simulink model "VCU_CS75_12_27_test"  (R2014a)
settings: Solver=FixedStepDiscrete  StartTime=0.0  StopTime=25  FixedStep=0.0005  RelTol=1e-3
undefined symbols (not defined in the file): D1, D2, D3, ecucoder_acal, ErrorSumMax1, ErrorSumMax2, ErrorSumMax3, I1, I2, I3, I_SW01_L, LaterlAngleCommand, LDW, P1, P2, P3, RemoteAcclPosition
libraries: simulink x913, ec5744lib x39
(part 19 of 30)

== system VCU_CS75_12_27_test/长安CS75底盘程序，20ms一次/Output/Subsystem/TransmitMessages1/ACC_34E/ACC_RLaneDistanceFusion ==
  ACC_RLaneDistanceFusion : Inport
  ACC_RLaneDistanceFusionBitCov : DataTypeConversion  OutDataTypeStr=uint8
  ACC_RLaneDistanceFusionCOV : DataTypeConversion  OutDataTypeStr=uint8
  ACC_RLaneDistanceFusionRon : Rounding  Operator=round
  ACC_RLaneDistanceFusion_1sat : Saturate  UpperLimit=1016  LowerLimit=0
  ACC_RLaneDistanceFusion_And : simulink/Logic and Bit Operations/Bitwise Operator  logicop=AND  UseBitMask=off  NumInputPorts=2  BitMask=bin2dec('11011001')  BitMaskRealWorld=Stored Integer
  ACC_RLaneDistanceFusion_And_C : Constant  Value=255  OutDataTypeStr=uint32
  ACC_RLaneDistanceFusion_Convert : DataTypeConversion  OutDataTypeStr=uint32
  ACC_RLaneDistanceFusion_D : Product  Inputs=*/
  ACC_RLaneDistanceFusion_D1 : Product  Inputs=*/
  ACC_RLaneDistanceFusion_F : Constant  Value=0.05  OutDataTypeStr=single
  ACC_RLaneDistanceFusion_L : simulink/Logic and Bit Operations/Bitwise Operator  logicop=AND  UseBitMask=on  BitMask=1016  BitMaskRealWorld=Stored Integer
  ACC_RLaneDistanceFusion_O : Constant  Value=0  OutDataTypeStr=single
  ACC_RLaneDistanceFusion_S : ArithShift  BitShiftNumber=-3
  ACC_RLaneDistanceFusion_sat : Saturate  UpperLimit=6.35  LowerLimit=0
  ACC_RLaneDistanceFusion_st : Sum  Inputs=+-
  ACC_RLaneDistanceFusionoutput2_C : Constant  Value=256
  Constant{1,4..8} (6 alike) : Constant  Value=0  OutDataTypeStr=uint8
  output1 : Outport
  output2 : Outport  Port=2
  output3 : Outport  Port=3
  output4 : Outport  Port=4
  output5 : Outport  Port=5
  output6 : Outport  Port=6
  output7 : Outport  Port=7
  output8 : Outport  Port=8
  wires:
  ACC_RLaneDistanceFusion/1 -> ACC_RLaneDistanceFusion_sat/1
  ACC_RLaneDistanceFusion_sat/1 -> ACC_RLaneDistanceFusion_st/1
  ACC_RLaneDistanceFusion_O/1 -> ACC_RLaneDistanceFusion_st/2
  ACC_RLaneDistanceFusion_st/1 -> ACC_RLaneDistanceFusion_D/1
  ACC_RLaneDistanceFusion_F/1 -> ACC_RLaneDistanceFusion_D/2
  ACC_RLaneDistanceFusion_D/1 -> ACC_RLaneDistanceFusionRon/1
  ACC_RLaneDistanceFusionRon/1 -> ACC_RLaneDistanceFusion_S/1
  ACC_RLaneDistanceFusion_S/1 -> ACC_RLaneDistanceFusion_1sat/1
  ACC_RLaneDistanceFusion_1sat/1 -> ACC_RLaneDistanceFusion_Convert/1
  ACC_RLaneDistanceFusion_Convert/1 -> ACC_RLaneDistanceFusion_L/1
  ACC_RLaneDistanceFusion_L/1 -> ACC_RLaneDistanceFusion_D1/1, ACC_RLaneDistanceFusion_And/1
  ACC_RLaneDistanceFusionoutput2_C/1 -> ACC_RLaneDistanceFusion_D1/2
  ACC_RLaneDistanceFusion_D1/1 -> ACC_RLaneDistanceFusionCOV/1
  ACC_RLaneDistanceFusionCOV/1 -> output2/1
  ACC_RLaneDistanceFusion_And_C/1 -> ACC_RLaneDistanceFusion_And/2
  ACC_RLaneDistanceFusion_And/1 -> ACC_RLaneDistanceFusionBitCov/1
  ACC_RLaneDistanceFusionBitCov/1 -> output3/1
  Constant1/1 -> output1/1
  Constant4/1 -> output4/1
  Constant5/1 -> output5/1
  Constant6/1 -> output6/1
  Constant7/1 -> output7/1
  Constant8/1 -> output8/1

== system VCU_CS75_12_27_test/长安CS75底盘程序，20ms一次/Output/Subsystem/TransmitMessages1/ACC_34E/ACC_RelevantTargetDection ==
  ACC_RelevantTargetDection : Inport
  ACC_RelevantTargetDectionRon : Rounding  Operator=round
  ACC_RelevantTargetDection_1sat : Saturate  UpperLimit=12  LowerLimit=0
  ACC_RelevantTargetDection_Convert : DataTypeConversion  OutDataTypeStr=uint8
  ACC_RelevantTargetDection_Convert1 : DataTypeConversion  OutDataTypeStr=uint32
  ACC_RelevantTargetDection_D : Product  Inputs=*/
  ACC_RelevantTargetDection_F : Constant  OutDataTypeStr=single
  ACC_RelevantTargetDection_L : simulink/Logic and Bit Operations/Bitwise Operator  logicop=AND  UseBitMask=on  BitMask=12  BitMaskRealWorld=Stored Integer
  ACC_RelevantTargetDection_O : Constant  Value=0  OutDataTypeStr=single
  ACC_RelevantTargetDection_S : ArithShift  BitShiftNumber=-2
  ACC_RelevantTargetDection_sat : Saturate  UpperLimit=3  LowerLimit=0
  ACC_RelevantTargetDection_st : Sum  Inputs=+-
  Constant{1,3..8} (7 alike) : Constant  Value=0  OutDataTypeStr=uint8
  output1 : Outport
  output2 : Outport  Port=2
  output3 : Outport  Port=3
  output4 : Outport  Port=4
  output5 : Outport  Port=5
  output6 : Outport  Port=6
  output7 : Outport  Port=7
  output8 : Outport  Port=8
  wires:
  ACC_RelevantTargetDection/1 -> ACC_RelevantTargetDection_sat/1
  ACC_RelevantTargetDection_sat/1 -> ACC_RelevantTargetDection_st/1
  ACC_RelevantTargetDection_O/1 -> ACC_RelevantTargetDection_st/2
  ACC_RelevantTargetDection_st/1 -> ACC_RelevantTargetDection_D/1
  ACC_RelevantTargetDection_F/1 -> ACC_RelevantTargetDection_D/2
  ACC_RelevantTargetDection_D/1 -> ACC_RelevantTargetDectionRon/1
  ACC_RelevantTargetDectionRon/1 -> ACC_RelevantTargetDection_S/1
  ACC_RelevantTargetDection_S/1 -> ACC_RelevantTargetDection_1sat/1
  ACC_RelevantTargetDection_1sat/1 -> ACC_RelevantTargetDection_Convert1/1
  ACC_RelevantTargetDection_Convert1/1 -> ACC_RelevantTargetDection_L/1
  ACC_RelevantTargetDection_L/1 -> ACC_RelevantTargetDection_Convert/1
  ACC_RelevantTargetDection_Convert/1 -> output2/1
  Constant1/1 -> output1/1
  Constant3/1 -> output3/1
  Constant4/1 -> output4/1
  Constant5/1 -> output5/1
  Constant6/1 -> output6/1
  Constant7/1 -> output7/1
  Constant8/1 -> output8/1

== system VCU_CS75_12_27_test/长安CS75底盘程序，20ms一次/Output/Subsystem/TransmitMessages1/ACC_34E/ACC_RelevantTargetID ==
  ACC_RelevantTargetID : Inport
  ACC_RelevantTargetIDRon : Rounding  Operator=round
  ACC_RelevantTargetID_1sat : Saturate  UpperLimit=240  LowerLimit=0
  ACC_RelevantTargetID_Convert : DataTypeConversion  OutDataTypeStr=uint8
  ACC_RelevantTargetID_Convert1 : DataTypeConversion  OutDataTypeStr=uint32
  ACC_RelevantTargetID_D : Product  Inputs=*/
  ACC_RelevantTargetID_F : Constant  OutDataTypeStr=single
  ACC_RelevantTargetID_L : simulink/Logic and Bit Operations/Bitwise Operator  logicop=AND  UseBitMask=on  BitMask=240  BitMaskRealWorld=Stored Integer
  ACC_RelevantTargetID_O : Constant  Value=0  OutDataTypeStr=single
  ACC_RelevantTargetID_S : ArithShift  BitShiftNumber=-4
  ACC_RelevantTargetID_sat : Saturate  UpperLimit=15  LowerLimit=0
  ACC_RelevantTargetID_st : Sum  Inputs=+-
  Constant{2..8} (7 alike) : Constant  Value=0  OutDataTypeStr=uint8
  output1 : Outport
  output2 : Outport  Port=2
  output3 : Outport  Port=3
  output4 : Outport  Port=4
  output5 : Outport  Port=5
  output6 : Outport  Port=6
  output7 : Outport  Port=7
  output8 : Outport  Port=8
  wires:
  ACC_RelevantTargetID/1 -> ACC_RelevantTargetID_sat/1
  ACC_RelevantTargetID_sat/1 -> ACC_RelevantTargetID_st/1
  ACC_RelevantTargetID_O/1 -> ACC_RelevantTargetID_st/2
  ACC_RelevantTargetID_st/1 -> ACC_RelevantTargetID_D/1
  ACC_RelevantTargetID_F/1 -> ACC_RelevantTargetID_D/2
  ACC_RelevantTargetID_D/1 -> ACC_RelevantTargetIDRon/1
  ACC_RelevantTargetIDRon/1 -> ACC_RelevantTargetID_S/1
  ACC_RelevantTargetID_S/1 -> ACC_RelevantTargetID_1sat/1
  ACC_RelevantTargetID_1sat/1 -> ACC_RelevantTargetID_Convert1/1
  ACC_RelevantTargetID_Convert1/1 -> ACC_RelevantTargetID_L/1
  ACC_RelevantTargetID_L/1 -> ACC_RelevantTargetID_Convert/1
  ACC_RelevantTargetID_Convert/1 -> output1/1
  Constant2/1 -> output2/1
  Constant3/1 -> output3/1
  Constant4/1 -> output4/1
  Constant5/1 -> output5/1
  Constant6/1 -> output6/1
  Constant7/1 -> output7/1
  Constant8/1 -> output8/1

== system VCU_CS75_12_27_test/长安CS75底盘程序，20ms一次/Output/Subsystem/TransmitMessages1/ACC_34E/ACC_RightTargetID ==
  ACC_RightTargetID : Inport
  ACC_RightTargetIDRon : Rounding  Operator=round
  ACC_RightTargetID_1sat : Saturate  UpperLimit=240  LowerLimit=0
  ACC_RightTargetID_Convert : DataTypeConversion  OutDataTypeStr=uint8
  ACC_RightTargetID_Convert1 : DataTypeConversion  OutDataTypeStr=uint32
  ACC_RightTargetID_D : Product  Inputs=*/
  ACC_RightTargetID_F : Constant  OutDataTypeStr=single
  ACC_RightTargetID_L : simulink/Logic and Bit Operations/Bitwise Operator  logicop=AND  UseBitMask=on  BitMask=240  BitMaskRealWorld=Stored Integer
  ACC_RightTargetID_O : Constant  Value=0  OutDataTypeStr=single
  ACC_RightTargetID_S : ArithShift  BitShiftNumber=-4
  ACC_RightTargetID_sat : Saturate  UpperLimit=15  LowerLimit=0
  ACC_RightTargetID_st : Sum  Inputs=+-
  Constant{1,3..8} (7 alike) : Constant  Value=0  OutDataTypeStr=uint8
  output1 : Outport
  output2 : Outport  Port=2
  output3 : Outport  Port=3
  output4 : Outport  Port=4
  output5 : Outport  Port=5
  output6 : Outport  Port=6
  output7 : Outport  Port=7
  output8 : Outport  Port=8
  wires:
  ACC_RightTargetID/1 -> ACC_RightTargetID_sat/1
  ACC_RightTargetID_sat/1 -> ACC_RightTargetID_st/1
  ACC_RightTargetID_O/1 -> ACC_RightTargetID_st/2
  ACC_RightTargetID_st/1 -> ACC_RightTargetID_D/1
  ACC_RightTargetID_F/1 -> ACC_RightTargetID_D/2
  ACC_RightTargetID_D/1 -> ACC_RightTargetIDRon/1
  ACC_RightTargetIDRon/1 -> ACC_RightTargetID_S/1
  ACC_RightTargetID_S/1 -> ACC_RightTargetID_1sat/1
  ACC_RightTargetID_1sat/1 -> ACC_RightTargetID_Convert1/1
  ACC_RightTargetID_Convert1/1 -> ACC_RightTargetID_L/1
  ACC_RightTargetID_L/1 -> ACC_RightTargetID_Convert/1
  ACC_RightTargetID_Convert/1 -> output2/1
  Constant1/1 -> output1/1
  Constant3/1 -> output3/1
  Constant4/1 -> output4/1
  Constant5/1 -> output5/1
  Constant6/1 -> output6/1
  Constant7/1 -> output7/1
  Constant8/1 -> output8/1

== system VCU_CS75_12_27_test/长安CS75底盘程序，20ms一次/Output/Subsystem/TransmitMessages10/LAS_29D/CRC ==
  CRC : Inport
  CRCRon : Rounding  Operator=round
  CRC_1sat : Saturate  UpperLimit=255  LowerLimit=0
  CRC_Convert : DataTypeConversion  OutDataTypeStr=uint8
  CRC_Convert1 : DataTypeConversion  OutDataTypeStr=uint32
  CRC_D : Product  Inputs=*/
  CRC_F : Constant  OutDataTypeStr=single
  CRC_L : simulink/Logic and Bit Operations/Bitwise Operator  logicop=AND  UseBitMask=on  BitMask=255  BitMaskRealWorld=Stored Integer
  CRC_O : Constant  Value=0  OutDataTypeStr=single
  CRC_S : ArithShift
  CRC_sat : Saturate  UpperLimit=0  LowerLimit=0
  CRC_st : Sum  Inputs=+-
  Constant{1..7} (7 alike) : Constant  Value=0  OutDataTypeStr=uint8
  output1 : Outport
  output2 : Outport  Port=2
  output3 : Outport  Port=3
  output4 : Outport  Port=4
  output5 : Outport  Port=5
  output6 : Outport  Port=6
  output7 : Outport  Port=7
  output8 : Outport  Port=8
  wires:
  CRC/1 -> CRC_sat/1
  CRC_sat/1 -> CRC_st/1
  CRC_O/1 -> CRC_st/2
  CRC_st/1 -> CRC_D/1
  CRC_F/1 -> CRC_D/2
  CRC_D/1 -> CRCRon/1
  CRCRon/1 -> CRC_S/1
  CRC_S/1 -> CRC_1sat/1
  CRC_1sat/1 -> CRC_Convert1/1
  CRC_Convert1/1 -> CRC_L/1
  CRC_L/1 -> CRC_Convert/1
  CRC_Convert/1 -> output8/1
  Constant1/1 -> output1/1
  Constant2/1 -> output2/1
  Constant3/1 -> output3/1
  Constant4/1 -> output4/1
  Constant5/1 -> output5/1
  Constant6/1 -> output6/1
  Constant7/1 -> output7/1

== system VCU_CS75_12_27_test/长安CS75底盘程序，20ms一次/Output/Subsystem/TransmitMessages10/LAS_29D/LAS_FatigueDectionEnableStatus ==
  LAS_FatigueDectionEnableStatus : Inport
  Constant{1,3..8} (7 alike) : Constant  Value=0  OutDataTypeStr=uint8
  LAS_FatigueDectionEnableStatusRon : Rounding  Operator=round
  LAS_FatigueDectionEnableStatus_1sat : Saturate  UpperLimit=12  LowerLimit=0
  LAS_FatigueDectionEnableStatus_Convert : DataTypeConversion  OutDataTypeStr=uint8
  LAS_FatigueDectionEnableStatus_Convert1 : DataTypeConversion  OutDataTypeStr=uint32
  LAS_FatigueDectionEnableStatus_D : Product  Inputs=*/
  LAS_FatigueDectionEnableStatus_F : Constant  OutDataTypeStr=single
  LAS_FatigueDectionEnableStatus_L : simulink/Logic and Bit Operations/Bitwise Operator  logicop=AND  UseBitMask=on  BitMask=12  BitMaskRealWorld=Stored Integer
  LAS_FatigueDectionEnableStatus_O : Constant  Value=0  OutDataTypeStr=single
  LAS_FatigueDectionEnableStatus_S : ArithShift  BitShiftNumber=-2
  LAS_FatigueDectionEnableStatus_sat : Saturate  UpperLimit=3  LowerLimit=0
  LAS_FatigueDectionEnableStatus_st : Sum  Inputs=+-
  output1 : Outport
  output2 : Outport  Port=2
  output3 : Outport  Port=3
  output4 : Outport  Port=4
  output5 : Outport  Port=5
  output6 : Outport  Port=6
  output7 : Outport  Port=7
  output8 : Outport  Port=8
  wires:
  LAS_FatigueDectionEnableStatus/1 -> LAS_FatigueDectionEnableStatus_sat/1
  LAS_FatigueDectionEnableStatus_sat/1 -> LAS_FatigueDectionEnableStatus_st/1
  LAS_FatigueDectionEnableStatus_O/1 -> LAS_FatigueDectionEnableStatus_st/2
  LAS_FatigueDectionEnableStatus_st/1 -> LAS_FatigueDectionEnableStatus_D/1
  LAS_FatigueDectionEnableStatus_F/1 -> LAS_FatigueDectionEnableStatus_D/2
  LAS_FatigueDectionEnableStatus_D/1 -> LAS_FatigueDectionEnableStatusRon/1
  LAS_FatigueDectionEnableStatusRon/1 -> LAS_FatigueDectionEnableStatus_S/1
  LAS_FatigueDectionEnableStatus_S/1 -> LAS_FatigueDectionEnableStatus_1sat/1
  LAS_FatigueDectionEnableStatus_1sat/1 -> LAS_FatigueDectionEnableStatus_Convert1/1
  LAS_FatigueDectionEnableStatus_Convert1/1 -> LAS_FatigueDectionEnableStatus_L/1
  LAS_FatigueDectionEnableStatus_L/1 -> LAS_FatigueDectionEnableStatus_Convert/1
  LAS_FatigueDectionEnableStatus_Convert/1 -> output2/1
  Constant1/1 -> output1/1
  Constant3/1 -> output3/1
  Constant4/1 -> output4/1
  Constant5/1 -> output5/1
  Constant6/1 -> output6/1
  Constant7/1 -> output7/1
  Constant8/1 -> output8/1

== system VCU_CS75_12_27_test/长安CS75底盘程序，20ms一次/Output/Subsystem/TransmitMessages10/LAS_29D/LAS_HMAEnableStatus ==
  LAS_HMAEnableStatus : Inport
  Constant{2..8} (7 alike) : Constant  Value=0  OutDataTypeStr=uint8
  LAS_HMAEnableStatusRon : Rounding  Operator=round
  LAS_HMAEnableStatus_1sat : Saturate  UpperLimit=4  LowerLimit=0
  LAS_HMAEnableStatus_Convert : DataTypeConversion  OutDataTypeStr=uint8
  LAS_HMAEnableStatus_Convert1 : DataTypeConversion  OutDataTypeStr=uint32
  LAS_HMAEnableStatus_D : Product  Inputs=*/
  LAS_HMAEnableStatus_F : Constant  OutDataTypeStr=single
  LAS_HMAEnableStatus_L : simulink/Logic and Bit Operations/Bitwise Operator  logicop=AND  UseBitMask=on  BitMask=4  BitMaskRealWorld=Stored Integer
  LAS_HMAEnableStatus_O : Constant  Value=0  OutDataTypeStr=single
  LAS_HMAEnableStatus_S : ArithShift  BitShiftNumber=-2
  LAS_HMAEnableStatus_sat : Saturate  UpperLimit=1  LowerLimit=0
  LAS_HMAEnableStatus_st : Sum  Inputs=+-
  output1 : Outport
  output2 : Outport  Port=2
  output3 : Outport  Port=3
  output4 : Outport  Port=4
  output5 : Outport  Port=5
  output6 : Outport  Port=6
  output7 : Outport  Port=7
  output8 : Outport  Port=8
  wires:
  LAS_HMAEnableStatus/1 -> LAS_HMAEnableStatus_sat/1
  LAS_HMAEnableStatus_sat/1 -> LAS_HMAEnableStatus_st/1
  LAS_HMAEnableStatus_O/1 -> LAS_HMAEnableStatus_st/2
  LAS_HMAEnableStatus_st/1 -> LAS_HMAEnableStatus_D/1
  LAS_HMAEnableStatus_F/1 -> LAS_HMAEnableStatus_D/2
  LAS_HMAEnableStatus_D/1 -> LAS_HMAEnableStatusRon/1
  LAS_HMAEnableStatusRon/1 -> LAS_HMAEnableStatus_S/1
  LAS_HMAEnableStatus_S/1 -> LAS_HMAEnableStatus_1sat/1
  LAS_HMAEnableStatus_1sat/1 -> LAS_HMAEnableStatus_Convert1/1
  LAS_HMAEnableStatus_Convert1/1 -> LAS_HMAEnableStatus_L/1
  LAS_HMAEnableStatus_L/1 -> LAS_HMAEnableStatus_Convert/1
  LAS_HMAEnableStatus_Convert/1 -> output1/1
  Constant2/1 -> output2/1
  Constant3/1 -> output3/1
  Constant4/1 -> output4/1
  Constant5/1 -> output5/1
  Constant6/1 -> output6/1
  Constant7/1 -> output7/1
  Constant8/1 -> output8/1

== system VCU_CS75_12_27_test/长安CS75底盘程序，20ms一次/Output/Subsystem/TransmitMessages10/LAS_29D/LAS_HostLaneLeftStatus ==
  LAS_HostLaneLeftStatus : Inport
  Constant{1..2,4..8} (7 alike) : Constant  Value=0  OutDataTypeStr=uint8
  LAS_HostLaneLeftStatusRon : Rounding  Operator=round
  LAS_HostLaneLeftStatus_1sat : Saturate  UpperLimit=7  LowerLimit=0
  LAS_HostLaneLeftStatus_Convert : DataTypeConversion  OutDataTypeStr=uint8
  LAS_HostLaneLeftStatus_Convert1 : DataTypeConversion  OutDataTypeStr=uint32
  LAS_HostLaneLeftStatus_D : Product  Inputs=*/
  LAS_HostLaneLeftStatus_F : Constant  OutDataTypeStr=single
  LAS_HostLaneLeftStatus_L : simulink/Logic and Bit Operations/Bitwise Operator  logicop=AND  UseBitMask=on  BitMask=7  BitMaskRealWorld=Stored Integer
  LAS_HostLaneLeftStatus_O : Constant  Value=0  OutDataTypeStr=single
  LAS_HostLaneLeftStatus_S : ArithShift
  LAS_HostLaneLeftStatus_sat : Saturate  UpperLimit=0  LowerLimit=0
  LAS_HostLaneLeftStatus_st : Sum  Inputs=+-
  output1 : Outport
  output2 : Outport  Port=2
  output3 : Outport  Port=3
  output4 : Outport  Port=4
  output5 : Outport  Port=5
  output6 : Outport  Port=6
  output7 : Outport  Port=7
  output8 : Outport  Port=8
  wires:
  LAS_HostLaneLeftStatus/1 -> LAS_HostLaneLeftStatus_sat/1
  LAS_HostLaneLeftStatus_sat/1 -> LAS_HostLaneLeftStatus_st/1
  LAS_HostLaneLeftStatus_O/1 -> LAS_HostLaneLeftStatus_st/2
  LAS_HostLaneLeftStatus_st/1 -> LAS_HostLaneLeftStatus_D/1
  LAS_HostLaneLeftStatus_F/1 -> LAS_HostLaneLeftStatus_D/2
  LAS_HostLaneLeftStatus_D/1 -> LAS_HostLaneLeftStatusRon/1
  LAS_HostLaneLeftStatusRon/1 -> LAS_HostLaneLeftStatus_S/1
  LAS_HostLaneLeftStatus_S/1 -> LAS_HostLaneLeftStatus_1sat/1
  LAS_HostLaneLeftStatus_1sat/1 -> LAS_HostLaneLeftStatus_Convert1/1
  LAS_HostLaneLeftStatus_Convert1/1 -> LAS_HostLaneLeftStatus_L/1
  LAS_HostLaneLeftStatus_L/1 -> LAS_HostLaneLeftStatus_Convert/1
  LAS_HostLaneLeftStatus_Convert/1 -> output3/1
  Constant1/1 -> output1/1
  Constant2/1 -> output2/1
  Constant4/1 -> output4/1
  Constant5/1 -> output5/1
  Constant6/1 -> output6/1
  Constant7/1 -> output7/1
  Constant8/1 -> output8/1

== system VCU_CS75_12_27_test/长安CS75底盘程序，20ms一次/Output/Subsystem/TransmitMessages10/LAS_29D/LAS_HostLaneRightStatus ==
  LAS_HostLaneRightStatus : Inport
  Constant{1..3,5..8} (7 alike) : Constant  Value=0  OutDataTypeStr=uint8
  LAS_HostLaneRightStatusRon : Rounding  Operator=round
  LAS_HostLaneRightStatus_1sat : Saturate  UpperLimit=7  LowerLimit=0
  LAS_HostLaneRightStatus_Convert : DataTypeConversion  OutDataTypeStr=uint8
  LAS_HostLaneRightStatus_Convert1 : DataTypeConversion  OutDataTypeStr=uint32
  LAS_HostLaneRightStatus_D : Product  Inputs=*/
  LAS_HostLaneRightStatus_F : Constant  OutDataTypeStr=single
  LAS_HostLaneRightStatus_L : simulink/Logic and Bit Operations/Bitwise Operator  logicop=AND  UseBitMask=on  BitMask=7  BitMaskRealWorld=Stored Integer
  LAS_HostLaneRightStatus_O : Constant  Value=0  OutDataTypeStr=single
  LAS_HostLaneRightStatus_S : ArithShift
  LAS_HostLaneRightStatus_sat : Saturate  UpperLimit=0  LowerLimit=0
  LAS_HostLaneRightStatus_st : Sum  Inputs=+-
  output1 : Outport
  output2 : Outport  Port=2
  output3 : Outport  Port=3
  output4 : Outport  Port=4
  output5 : Outport  Port=5
  output6 : Outport  Port=6
  output7 : Outport  Port=7
  output8 : Outport  Port=8
  wires:
  LAS_HostLaneRightStatus/1 -> LAS_HostLaneRightStatus_sat/1
  LAS_HostLaneRightStatus_sat/1 -> LAS_HostLaneRightStatus_st/1
  LAS_HostLaneRightStatus_O/1 -> LAS_HostLaneRightStatus_st/2
  LAS_HostLaneRightStatus_st/1 -> LAS_HostLaneRightStatus_D/1
  LAS_HostLaneRightStatus_F/1 -> LAS_HostLaneRightStatus_D/2
  LAS_HostLaneRightStatus_D/1 -> LAS_HostLaneRightStatusRon/1
  LAS_HostLaneRightStatusRon/1 -> LAS_HostLaneRightStatus_S/1
  LAS_HostLaneRightStatus_S/1 -> LAS_HostLaneRightStatus_1sat/1
  LAS_HostLaneRightStatus_1sat/1 -> LAS_HostLaneRightStatus_Convert1/1
  LAS_HostLaneRightStatus_Convert1/1 -> LAS_HostLaneRightStatus_L/1
  LAS_HostLaneRightStatus_L/1 -> LAS_HostLaneRightStatus_Convert/1
  LAS_HostLaneRightStatus_Convert/1 -> output4/1
  Constant1/1 -> output1/1
  Constant2/1 -> output2/1
  Constant3/1 -> output3/1
  Constant5/1 -> output5/1
  Constant6/1 -> output6/1
  Constant7/1 -> output7/1
  Constant8/1 -> output8/1

== system VCU_CS75_12_27_test/长安CS75底盘程序，20ms一次/Output/Subsystem/TransmitMessages10/LAS_29D/LAS_IACCEnableStatus ==
  LAS_IACCEnableStatus : Inport
  Constant{1..6,8} (7 alike) : Constant  Value=0  OutDataTypeStr=uint8
  LAS_IACCEnableStatusRon : Rounding  Operator=round
  LAS_IACCEnableStatus_1sat : Saturate  UpperLimit=48  LowerLimit=0
  LAS_IACCEnableStatus_Convert : DataTypeConversion  OutDataTypeStr=uint8
  LAS_IACCEnableStatus_Convert1 : DataTypeConversion  OutDataTypeStr=uint32
  LAS_IACCEnableStatus_D : Product  Inputs=*/
  LAS_IACCEnableStatus_F : Constant  OutDataTypeStr=single
  LAS_IACCEnableStatus_L : simulink/Logic and Bit Operations/Bitwise Operator  logicop=AND  UseBitMask=on  BitMask=48  BitMaskRealWorld=Stored Integer
  LAS_IACCEnableStatus_O : Constant  Value=0  OutDataTypeStr=single
  LAS_IACCEnableStatus_S : ArithShift  BitShiftNumber=-4
  LAS_IACCEnableStatus_sat : Saturate  UpperLimit=3  LowerLimit=0
  LAS_IACCEnableStatus_st : Sum  Inputs=+-
  output1 : Outport
  output2 : Outport  Port=2
  output3 : Outport  Port=3
  output4 : Outport  Port=4
  output5 : Outport  Port=5
  output6 : Outport  Port=6
  output7 : Outport  Port=7
  output8 : Outport  Port=8
  wires:
  LAS_IACCEnableStatus/1 -> LAS_IACCEnableStatus_sat/1
  LAS_IACCEnableStatus_sat/1 -> LAS_IACCEnableStatus_st/1
  LAS_IACCEnableStatus_O/1 -> LAS_IACCEnableStatus_st/2
  LAS_IACCEnableStatus_st/1 -> LAS_IACCEnableStatus_D/1
  LAS_IACCEnableStatus_F/1 -> LAS_IACCEnableStatus_D/2
  LAS_IACCEnableStatus_D/1 -> LAS_IACCEnableStatusRon/1
  LAS_IACCEnableStatusRon/1 -> LAS_IACCEnableStatus_S/1
  LAS_IACCEnableStatus_S/1 -> LAS_IACCEnableStatus_1sat/1
  LAS_IACCEnableStatus_1sat/1 -> LAS_IACCEnableStatus_Convert1/1
  LAS_IACCEnableStatus_Convert1/1 -> LAS_IACCEnableStatus_L/1
  LAS_IACCEnableStatus_L/1 -> LAS_IACCEnableStatus_Convert/1
  LAS_IACCEnableStatus_Convert/1 -> output7/1
  Constant1/1 -> output1/1
  Constant2/1 -> output2/1
  Constant3/1 -> output3/1
  Constant4/1 -> output4/1
  Constant5/1 -> output5/1
  Constant6/1 -> output6/1
  Constant8/1 -> output8/1

== system VCU_CS75_12_27_test/长安CS75底盘程序，20ms一次/Output/Subsystem/TransmitMessages10/LAS_29D/LAS_LASModeSelectionStatus ==
  LAS_LASModeSelectionStatus : Inport
  Constant{2..8} (7 alike) : Constant  Value=0  OutDataTypeStr=uint8
  LAS_LASModeSelectionStatusRon : Rounding  Operator=round
  LAS_LASModeSelectionStatus_1sat : Saturate  UpperLimit=56  LowerLimit=0
  LAS_LASModeSelectionStatus_Convert : DataTypeConversion  OutDataTypeStr=uint8
  LAS_LASModeSelectionStatus_Convert1 : DataTypeConversion  OutDataTypeStr=uint32
  LAS_LASModeSelectionStatus_D : Product  Inputs=*/
  LAS_LASModeSelectionStatus_F : Constant  OutDataTypeStr=single
  LAS_LASModeSelectionStatus_L : simulink/Logic and Bit Operations/Bitwise Operator  logicop=AND  UseBitMask=on  BitMask=56  BitMaskRealWorld=Stored Integer
  LAS_LASModeSelectionStatus_O : Constant  Value=0  OutDataTypeStr=single
  LAS_LASModeSelectionStatus_S : ArithShift  BitShiftNumber=-3
  LAS_LASModeSelectionStatus_sat : Saturate  UpperLimit=7  LowerLimit=0
  LAS_LASModeSelectionStatus_st : Sum  Inputs=+-
  output1 : Outport
  output2 : Outport  Port=2
  output3 : Outport  Port=3
  output4 : Outport  Port=4
  output5 : Outport  Port=5
  output6 : Outport  Port=6
  output7 : Outport  Port=7
  output8 : Outport  Port=8
  wires:
  LAS_LASModeSelectionStatus/1 -> LAS_LASModeSelectionStatus_sat/1
  LAS_LASModeSelectionStatus_sat/1 -> LAS_LASModeSelectionStatus_st/1
  LAS_LASModeSelectionStatus_O/1 -> LAS_LASModeSelectionStatus_st/2
  LAS_LASModeSelectionStatus_st/1 -> LAS_LASModeSelectionStatus_D/1
  LAS_LASModeSelectionStatus_F/1 -> LAS_LASModeSelectionStatus_D/2
  LAS_LASModeSelectionStatus_D/1 -> LAS_LASModeSelectionStatusRon/1
  LAS_LASModeSelectionStatusRon/1 -> LAS_LASModeSelectionStatus_S/1
  LAS_LASModeSelectionStatus_S/1 -> LAS_LASModeSelectionStatus_1sat/1
  LAS_LASModeSelectionStatus_1sat/1 -> LAS_LASModeSelectionStatus_Convert1/1
  LAS_LASModeSelectionStatus_Convert1/1 -> LAS_LASModeSelectionStatus_L/1
  LAS_LASModeSelectionStatus_L/1 -> LAS_LASModeSelectionStatus_Convert/1
  LAS_LASModeSelectionStatus_Convert/1 -> output1/1
  Constant2/1 -> output2/1
  Constant3/1 -> output3/1
  Constant4/1 -> output4/1
  Constant5/1 -> output5/1
  Constant6/1 -> output6/1
  Constant7/1 -> output7/1
  Constant8/1 -> output8/1

== system VCU_CS75_12_27_test/长安CS75底盘程序，20ms一次/Output/Subsystem/TransmitMessages10/LAS_29D/LAS_LASWarningModeSelectionSts ==
  LAS_LASWarningModeSelectionSts : Inport
  Constant{3..8} (6 alike) : Constant  Value=0  OutDataTypeStr=uint8
  LAS_LASWarningModeSelectionStsBitCov : DataTypeConversion  OutDataTypeStr=uint8
  LAS_LASWarningModeSelectionStsCOV : DataTypeConversion  OutDataTypeStr=uint8
  LAS_LASWarningModeSelectionStsRon : Rounding  Operator=round
  LAS_LASWarningModeSelectionSts_1sat : Saturate  UpperLimit=448  LowerLimit=0
  LAS_LASWarningModeSelectionSts_And : simulink/Logic and Bit Operations/Bitwise Operator  logicop=AND  UseBitMask=off  NumInputPorts=2  BitMask=bin2dec('11011001')  BitMaskRealWorld=Stored Integer
  LAS_LASWarningModeSelectionSts_And_C : Constant  Value=255  OutDataTypeStr=uint32
  LAS_LASWarningModeSelectionSts_Convert : DataTypeConversion  OutDataTypeStr=uint32
  LAS_LASWarningModeSelectionSts_D : Product  Inputs=*/
  LAS_LASWarningModeSelectionSts_D1 : Product  Inputs=*/
  LAS_LASWarningModeSelectionSts_F : Constant  OutDataTypeStr=single
  LAS_LASWarningModeSelectionSts_L : simulink/Logic and Bit Operations/Bitwise Operator  logicop=AND  UseBitMask=on  BitMask=448  BitMaskRealWorld=Stored Integer
  LAS_LASWarningModeSelectionSts_O : Constant  Value=0  OutDataTypeStr=single
  LAS_LASWarningModeSelectionSts_S : ArithShift  BitShiftNumber=-6
  LAS_LASWarningModeSelectionSts_sat : Saturate  UpperLimit=7  LowerLimit=0
  LAS_LASWarningModeSelectionSts_st : Sum  Inputs=+-
  LAS_LASWarningModeSelectionStsoutput1_C : Constant  Value=256
  output1 : Outport
  output2 : Outport  Port=2
  output3 : Outport  Port=3
  output4 : Outport  Port=4
  output5 : Outport  Port=5
  output6 : Outport  Port=6
  output7 : Outport  Port=7
  output8 : Outport  Port=8
  wires:
  LAS_LASWarningModeSelectionSts/1 -> LAS_LASWarningModeSelectionSts_sat/1
  LAS_LASWarningModeSelectionSts_sat/1 -> LAS_LASWarningModeSelectionSts_st/1
  LAS_LASWarningModeSelectionSts_O/1 -> LAS_LASWarningModeSelectionSts_st/2
  LAS_LASWarningModeSelectionSts_st/1 -> LAS_LASWarningModeSelectionSts_D/1
  LAS_LASWarningModeSelectionSts_F/1 -> LAS_LASWarningModeSelectionSts_D/2
  LAS_LASWarningModeSelectionSts_D/1 -> LAS_LASWarningModeSelectionStsRon/1
  LAS_LASWarningModeSelectionStsRon/1 -> LAS_LASWarningModeSelectionSts_S/1
  LAS_LASWarningModeSelectionSts_S/1 -> LAS_LASWarningModeSelectionSts_1sat/1
  LAS_LASWarningModeSelectionSts_1sat/1 -> LAS_LASWarningModeSelectionSts_Convert/1
  LAS_LASWarningModeSelectionSts_Convert/1 -> LAS_LASWarningModeSelectionSts_L/1
  LAS_LASWarningModeSelectionSts_L/1 -> LAS_LASWarningModeSelectionSts_D1/1, LAS_LASWarningModeSelectionSts_And/1
  LAS_LASWarningModeSelectionStsoutput1_C/1 -> LAS_LASWarningModeSelectionSts_D1/2
  LAS_LASWarningModeSelectionSts_D1/1 -> LAS_LASWarningModeSelectionStsCOV/1
  LAS_LASWarningModeSelectionStsCOV/1 -> output1/1
  LAS_LASWarningModeSelectionSts_And_C/1 -> LAS_LASWarningModeSelectionSts_And/2
  LAS_LASWarningModeSelectionSts_And/1 -> LAS_LASWarningModeSelectionStsBitCov/1
  LAS_LASWarningModeSelectionStsBitCov/1 -> output2/1
  Constant3/1 -> output3/1
  Constant4/1 -> output4/1
  Constant5/1 -> output5/1
  Constant6/1 -> output6/1
  Constant7/1 -> output7/1
  Constant8/1 -> output8/1

== system VCU_CS75_12_27_test/长安CS75底盘程序，20ms一次/Output/Subsystem/TransmitMessages10/LAS_29D/LAS_LDWShakeLevStatus ==
  LAS_LDWShakeLevStatus : Inport
  Constant{1,3..8} (7 alike) : Constant  Value=0  OutDataTypeStr=uint8
  LAS_LDWShakeLevStatusRon : Rounding  Operator=round
  LAS_LDWShakeLevStatus_1sat : Saturate  UpperLimit=48  LowerLimit=0
  LAS_LDWShakeLevStatus_Convert : DataTypeConversion  OutDataTypeStr=uint8
  LAS_LDWShakeLevStatus_Convert1 : DataTypeConversion  OutDataTypeStr=uint32
  LAS_LDWShakeLevStatus_D : Product  Inputs=*/
  LAS_LDWShakeLevStatus_F : Constant  OutDataTypeStr=single
  LAS_LDWShakeLevStatus_L : simulink/Logic and Bit Operations/Bitwise Operator  logicop=AND  UseBitMask=on  BitMask=48  BitMaskRealWorld=Stored Integer
  LAS_LDWShakeLevStatus_O : Constant  Value=0  OutDataTypeStr=single
  LAS_LDWShakeLevStatus_S : ArithShift  BitShiftNumber=-4
  LAS_LDWShakeLevStatus_sat : Saturate  UpperLimit=3  LowerLimit=0
  LAS_LDWShakeLevStatus_st : Sum  Inputs=+-
  output1 : Outport
  output2 : Outport  Port=2
  output3 : Outport  Port=3
  output4 : Outport  Port=4
  output5 : Outport  Port=5
  output6 : Outport  Port=6
  output7 : Outport  Port=7
  output8 : Outport  Port=8
  wires:
  LAS_LDWShakeLevStatus/1 -> LAS_LDWShakeLevStatus_sat/1
  LAS_LDWShakeLevStatus_sat/1 -> LAS_LDWShakeLevStatus_st/1
  LAS_LDWShakeLevStatus_O/1 -> LAS_LDWShakeLevStatus_st/2
  LAS_LDWShakeLevStatus_st/1 -> LAS_LDWShakeLevStatus_D/1
  LAS_LDWShakeLevStatus_F/1 -> LAS_LDWShakeLevStatus_D/2
  LAS_LDWShakeLevStatus_D/1 -> LAS_LDWShakeLevStatusRon/1
  LAS_LDWShakeLevStatusRon/1 -> LAS_LDWShakeLevStatus_S/1
  LAS_LDWShakeLevStatus_S/1 -> LAS_LDWShakeLevStatus_1sat/1
  LAS_LDWShakeLevStatus_1sat/1 -> LAS_LDWShakeLevStatus_Convert1/1
  LAS_LDWShakeLevStatus_Convert1/1 -> LAS_LDWShakeLevStatus_L/1
  LAS_LDWShakeLevStatus_L/1 -> LAS_LDWShakeLevStatus_Convert/1
  LAS_LDWShakeLevStatus_Convert/1 -> output2/1
  Constant1/1 -> output1/1
  Constant3/1 -> output3/1
  Constant4/1 -> output4/1
  Constant5/1 -> output5/1
  Constant6/1 -> output6/1
  Constant7/1 -> output7/1
  Constant8/1 -> output8/1

== system VCU_CS75_12_27_test/长安CS75底盘程序，20ms一次/Output/Subsystem/TransmitMessages10/LAS_29D/LAS_LLaneMarkerType ==
  LAS_LLaneMarkerType : Inport
  Constant{1..4,6..8} (7 alike) : Constant  Value=0  OutDataTypeStr=uint8
  LAS_LLaneMarkerTypeRon : Rounding  Operator=round
  LAS_LLaneMarkerType_1sat : Saturate  UpperLimit=7  LowerLimit=0
  LAS_LLaneMarkerType_Convert : DataTypeConversion  OutDataTypeStr=uint8
  LAS_LLaneMarkerType_Convert1 : DataTypeConversion  OutDataTypeStr=uint32
  LAS_LLaneMarkerType_D : Product  Inputs=*/
  LAS_LLaneMarkerType_F : Constant  OutDataTypeStr=single
  LAS_LLaneMarkerType_L : simulink/Logic and Bit Operations/Bitwise Operator  logicop=AND  UseBitMask=on  BitMask=7  BitMaskRealWorld=Stored Integer
  LAS_LLaneMarkerType_O : Constant  Value=0  OutDataTypeStr=single
  LAS_LLaneMarkerType_S : ArithShift
  LAS_LLaneMarkerType_sat : Saturate  UpperLimit=7  LowerLimit=0
  LAS_LLaneMarkerType_st : Sum  Inputs=+-
  output1 : Outport
  output2 : Outport  Port=2
  output3 : Outport  Port=3
  output4 : Outport  Port=4
  output5 : Outport  Port=5
  output6 : Outport  Port=6
  output7 : Outport  Port=7
  output8 : Outport  Port=8
  wires:
  LAS_LLaneMarkerType/1 -> LAS_LLaneMarkerType_sat/1
  LAS_LLaneMarkerType_sat/1 -> LAS_LLaneMarkerType_st/1
  LAS_LLaneMarkerType_O/1 -> LAS_LLaneMarkerType_st/2
  LAS_LLaneMarkerType_st/1 -> LAS_LLaneMarkerType_D/1
  LAS_LLaneMarkerType_F/1 -> LAS_LLaneMarkerType_D/2
  LAS_LLaneMarkerType_D/1 -> LAS_LLaneMarkerTypeRon/1
  LAS_LLaneMarkerTypeRon/1 -> LAS_LLaneMarkerType_S/1
  LAS_LLaneMarkerType_S/1 -> LAS_LLaneMarkerType_1sat/1
  LAS_LLaneMarkerType_1sat/1 -> LAS_LLaneMarkerType_Convert1/1
  LAS_LLaneMarkerType_Convert1/1 -> LAS_LLaneMarkerType_L/1
  LAS_LLaneMarkerType_L/1 -> LAS_LLaneMarkerType_Convert/1
  LAS_LLaneMarkerType_Convert/1 -> output5/1
  Constant1/1 -> output1/1
  Constant2/1 -> output2/1
  Constant3/1 -> output3/1
  Constant4/1 -> output4/1
  Constant6/1 -> output6/1
  Constant7/1 -> output7/1
  Constant8/1 -> output8/1

== system VCU_CS75_12_27_test/长安CS75底盘程序，20ms一次/Output/Subsystem/TransmitMessages10/LAS_29D/LAS_LdwSensitivityStatus ==
  LAS_LdwSensitivityStatus : Inport
  Constant{2..8} (7 alike) : Constant  Value=0  OutDataTypeStr=uint8
  LAS_LdwSensitivityStatusRon : Rounding  Operator=round
  LAS_LdwSensitivityStatus_1sat : Saturate  UpperLimit=192  LowerLimit=0
  LAS_LdwSensitivityStatus_Convert : DataTypeConversion  OutDataTypeStr=uint8
  LAS_LdwSensitivityStatus_Convert1 : DataTypeConversion  OutDataTypeStr=uint32
  LAS_LdwSensitivityStatus_D : Product  Inputs=*/
  LAS_LdwSensitivityStatus_F : Constant  OutDataTypeStr=single
  LAS_LdwSensitivityStatus_L : simulink/Logic and Bit Operations/Bitwise Operator  logicop=AND  UseBitMask=on  BitMask=192  BitMaskRealWorld=Stored Integer
  LAS_LdwSensitivityStatus_O : Constant  Value=0  OutDataTypeStr=single
  LAS_LdwSensitivityStatus_S : ArithShift  BitShiftNumber=-6
  LAS_LdwSensitivityStatus_sat : Saturate  UpperLimit=3  LowerLimit=0
  LAS_LdwSensitivityStatus_st : Sum  Inputs=+-
  output1 : Outport
  output2 : Outport  Port=2
  output3 : Outport  Port=3
  output4 : Outport  Port=4
  output5 : Outport  Port=5
  output6 : Outport  Port=6
  output7 : Outport  Port=7
  output8 : Outport  Port=8
  wires:
  LAS_LdwSensitivityStatus/1 -> LAS_LdwSensitivityStatus_sat/1
  LAS_LdwSensitivityStatus_sat/1 -> LAS_LdwSensitivityStatus_st/1
  LAS_LdwSensitivityStatus_O/1 -> LAS_LdwSensitivityStatus_st/2
  LAS_LdwSensitivityStatus_st/1 -> LAS_LdwSensitivityStatus_D/1
  LAS_LdwSensitivityStatus_F/1 -> LAS_LdwSensitivityStatus_D/2
  LAS_LdwSensitivityStatus_D/1 -> LAS_LdwSensitivityStatusRon/1
  LAS_LdwSensitivityStatusRon/1 -> LAS_LdwSensitivityStatus_S/1
  LAS_LdwSensitivityStatus_S/1 -> LAS_LdwSensitivityStatus_1sat/1
  LAS_LdwSensitivityStatus_1sat/1 -> LAS_LdwSensitivityStatus_Convert1/1
  LAS_LdwSensitivityStatus_Convert1/1 -> LAS_LdwSensitivityStatus_L/1
  LAS_LdwSensitivityStatus_L/1 -> LAS_LdwSensitivityStatus_Convert/1
  LAS_LdwSensitivityStatus_Convert/1 -> output1/1
  Constant2/1 -> output2/1
  Constant3/1 -> output3/1
  Constant4/1 -> output4/1
  Constant5/1 -> output5/1
  Constant6/1 -> output6/1
  Constant7/1 -> output7/1
  Constant8/1 -> output8/1

== system VCU_CS75_12_27_test/长安CS75底盘程序，20ms一次/Output/Subsystem/TransmitMessages10/LAS_29D/LAS_OverspeedSoundWarning ==
  LAS_OverspeedSoundWarning : Inport
  Constant{1..3,5..8} (7 alike) : Constant  Value=0  OutDataTypeStr=uint8
  LAS_OverspeedSoundWarningRon : Rounding  Operator=round
  LAS_OverspeedSoundWarning_1sat : Saturate  UpperLimit=192  LowerLimit=0
  LAS_OverspeedSoundWarning_Convert : DataTypeConversion  OutDataTypeStr=uint8
  LAS_OverspeedSoundWarning_Convert1 : DataTypeConversion  OutDataTypeStr=uint32
  LAS_OverspeedSoundWarning_D : Product  Inputs=*/
  LAS_OverspeedSoundWarning_F : Constant  OutDataTypeStr=single
  LAS_OverspeedSoundWarning_L : simulink/Logic and Bit Operations/Bitwise Operator  logicop=AND  UseBitMask=on  BitMask=192  BitMaskRealWorld=Stored Integer
  LAS_OverspeedSoundWarning_O : Constant  Value=0  OutDataTypeStr=single
  LAS_OverspeedSoundWarning_S : ArithShift  BitShiftNumber=-6
  LAS_OverspeedSoundWarning_sat : Saturate  UpperLimit=3  LowerLimit=0
  LAS_OverspeedSoundWarning_st : Sum  Inputs=+-
  output1 : Outport
  output2 : Outport  Port=2
  output3 : Outport  Port=3
  output4 : Outport  Port=4
  output5 : Outport  Port=5
  output6 : Outport  Port=6
  output7 : Outport  Port=7
  output8 : Outport  Port=8
  wires:
  LAS_OverspeedSoundWarning/1 -> LAS_OverspeedSoundWarning_sat/1
  LAS_OverspeedSoundWarning_sat/1 -> LAS_OverspeedSoundWarning_st/1
  LAS_OverspeedSoundWarning_O/1 -> LAS_OverspeedSoundWarning_st/2
  LAS_OverspeedSoundWarning_st/1 -> LAS_OverspeedSoundWarning_D/1
  LAS_OverspeedSoundWarning_F/1 -> LAS_OverspeedSoundWarning_D/2
  LAS_OverspeedSoundWarning_D/1 -> LAS_OverspeedSoundWarningRon/1
  LAS_OverspeedSoundWarningRon/1 -> LAS_OverspeedSoundWarning_S/1
  LAS_OverspeedSoundWarning_S/1 -> LAS_OverspeedSoundWarning_1sat/1
  LAS_OverspeedSoundWarning_1sat/1 -> LAS_OverspeedSoundWarning_Convert1/1
  LAS_OverspeedSoundWarning_Convert1/1 -> LAS_OverspeedSoundWarning_L/1
  LAS_OverspeedSoundWarning_L/1 -> LAS_OverspeedSoundWarning_Convert/1
  LAS_OverspeedSoundWarning_Convert/1 -> output4/1
  Constant1/1 -> output1/1
  Constant2/1 -> output2/1
  Constant3/1 -> output3/1
  Constant5/1 -> output5/1
  Constant6/1 -> output6/1
  Constant7/1 -> output7/1
  Constant8/1 -> output8/1

== system VCU_CS75_12_27_test/长安CS75底盘程序，20ms一次/Output/Subsystem/TransmitMessages10/LAS_29D/LAS_OverspeedSoundWarningEnSt ==
  LAS_OverspeedSoundWarningEnSt : Inport
  Constant{1,3..8} (7 alike) : Constant  Value=0  OutDataTypeStr=uint8
  LAS_OverspeedSoundWarningEnStRon : Rounding  Operator=round
  LAS_OverspeedSoundWarningEnSt_1sat : Saturate  UpperLimit=3  LowerLimit=0
  LAS_OverspeedSoundWarningEnSt_Convert : DataTypeConversion  OutDataTypeStr=uint8
  LAS_OverspeedSoundWarningEnSt_Convert1 : DataTypeConversion  OutDataTypeStr=uint32
  LAS_OverspeedSoundWarningEnSt_D : Product  Inputs=*/
  LAS_OverspeedSoundWarningEnSt_F : Constant  OutDataTypeStr=single
  LAS_OverspeedSoundWarningEnSt_L : simulink/Logic and Bit Operations/Bitwise Operator  logicop=AND  UseBitMask=on  BitMask=3  BitMaskRealWorld=Stored Integer
  LAS_OverspeedSoundWarningEnSt_O : Constant  Value=0  OutDataTypeStr=single
  LAS_OverspeedSoundWarningEnSt_S : ArithShift
  LAS_OverspeedSoundWarningEnSt_sat : Saturate  UpperLimit=3  LowerLimit=0
  LAS_OverspeedSoundWarningEnSt_st : Sum  Inputs=+-
  output1 : Outport
  output2 : Outport  Port=2
  output3 : Outport  Port=3
  output4 : Outport  Port=4
  output5 : Outport  Port=5
  output6 : Outport  Port=6
  output7 : Outport  Port=7
  output8 : Outport  Port=8
  wires:
  LAS_OverspeedSoundWarningEnSt/1 -> LAS_OverspeedSoundWarningEnSt_sat/1
  LAS_OverspeedSoundWarningEnSt_sat/1 -> LAS_OverspeedSoundWarningEnSt_st/1
  LAS_OverspeedSoundWarningEnSt_O/1 -> LAS_OverspeedSoundWarningEnSt_st/2
  LAS_OverspeedSoundWarningEnSt_st/1 -> LAS_OverspeedSoundWarningEnSt_D/1
  LAS_OverspeedSoundWarningEnSt_F/1 -> LAS_OverspeedSoundWarningEnSt_D/2
  LAS_OverspeedSoundWarningEnSt_D/1 -> LAS_OverspeedSoundWarningEnStRon/1
  LAS_OverspeedSoundWarningEnStRon/1 -> LAS_OverspeedSoundWarningEnSt_S/1
  LAS_OverspeedSoundWarningEnSt_S/1 -> LAS_OverspeedSoundWarningEnSt_1sat/1
  LAS_OverspeedSoundWarningEnSt_1sat/1 -> LAS_OverspeedSoundWarningEnSt_Convert1/1
  LAS_OverspeedSoundWarningEnSt_Convert1/1 -> LAS_OverspeedSoundWarningEnSt_L/1
  LAS_OverspeedSoundWarningEnSt_L/1 -> LAS_OverspeedSoundWarningEnSt_Convert/1
  LAS_OverspeedSoundWarningEnSt_Convert/1 -> output2/1
  Constant1/1 -> output1/1
  Constant3/1 -> output3/1
  Constant4/1 -> output4/1
  Constant5/1 -> output5/1
  Constant6/1 -> output6/1
  Constant7/1 -> output7/1
  Constant8/1 -> output8/1

== system VCU_CS75_12_27_test/长安CS75底盘程序，20ms一次/Output/Subsystem/TransmitMessages10/LAS_29D/LAS_OverspeedVisualWarning ==
  LAS_OverspeedVisualWarning : Inport
  Constant{1..4,6..8} (7 alike) : Constant  Value=0  OutDataTypeStr=uint8
  LAS_OverspeedVisualWarningRon : Rounding  Operator=round
  LAS_OverspeedVisualWarning_1sat : Saturate  UpperLimit=192  LowerLimit=0
  LAS_OverspeedVisualWarning_Convert : DataTypeConversion  OutDataTypeStr=uint8
  LAS_OverspeedVisualWarning_Convert1 : DataTypeConversion  OutDataTypeStr=uint32
  LAS_OverspeedVisualWarning_D : Product  Inputs=*/
  LAS_OverspeedVisualWarning_F : Constant  OutDataTypeStr=single
  LAS_OverspeedVisualWarning_L : simulink/Logic and Bit Operations/Bitwise Operator  logicop=AND  UseBitMask=on  BitMask=192  BitMaskRealWorld=Stored Integer
  LAS_OverspeedVisualWarning_O : Constant  Value=0  OutDataTypeStr=single
  LAS_OverspeedVisualWarning_S : ArithShift  BitShiftNumber=-6
  LAS_OverspeedVisualWarning_sat : Saturate  UpperLimit=3  LowerLimit=0
  LAS_OverspeedVisualWarning_st : Sum  Inputs=+-
  output1 : Outport
  output2 : Outport  Port=2
  output3 : Outport  Port=3
  output4 : Outport  Port=4
  output5 : Outport  Port=5
  output6 : Outport  Port=6
  output7 : Outport  Port=7
  output8 : Outport  Port=8
  wires:
  LAS_OverspeedVisualWarning/1 -> LAS_OverspeedVisualWarning_sat/1
  LAS_OverspeedVisualWarning_sat/1 -> LAS_OverspeedVisualWarning_st/1
  LAS_OverspeedVisualWarning_O/1 -> LAS_OverspeedVisualWarning_st/2
  LAS_OverspeedVisualWarning_st/1 -> LAS_OverspeedVisualWarning_D/1
  LAS_OverspeedVisualWarning_F/1 -> LAS_OverspeedVisualWarning_D/2
  LAS_OverspeedVisualWarning_D/1 -> LAS_OverspeedVisualWarningRon/1
  LAS_OverspeedVisualWarningRon/1 -> LAS_OverspeedVisualWarning_S/1
  LAS_OverspeedVisualWarning_S/1 -> LAS_OverspeedVisualWarning_1sat/1
  LAS_OverspeedVisualWarning_1sat/1 -> LAS_OverspeedVisualWarning_Convert1/1
  LAS_OverspeedVisualWarning_Convert1/1 -> LAS_OverspeedVisualWarning_L/1
  LAS_OverspeedVisualWarning_L/1 -> LAS_OverspeedVisualWarning_Convert/1
  LAS_OverspeedVisualWarning_Convert/1 -> output5/1
  Constant1/1 -> output1/1
  Constant2/1 -> output2/1
  Constant3/1 -> output3/1
  Constant4/1 -> output4/1
  Constant6/1 -> output6/1
  Constant7/1 -> output7/1
  Constant8/1 -> output8/1

== system VCU_CS75_12_27_test/长安CS75底盘程序，20ms一次/Output/Subsystem/TransmitMessages10/LAS_29D/LAS_OverspeedWarningEnableStatus ==
  LAS_OverspeedWarningEnableStatus : Inport
  Constant{1..3,5..8} (7 alike) : Constant  Value=0  OutDataTypeStr=uint8
  LAS_OverspeedWarningEnableStatusRon : Rounding  Operator=round
  LAS_OverspeedWarningEnableStatus_1sat : Saturate  UpperLimit=48  LowerLimit=0
  LAS_OverspeedWarningEnableStatus_Convert : DataTypeConversion  OutDataTypeStr=uint8
  LAS_OverspeedWarningEnableStatus_Convert1 : DataTypeConversion  OutDataTypeStr=uint32
  LAS_OverspeedWarningEnableStatus_D : Product  Inputs=*/
  LAS_OverspeedWarningEnableStatus_F : Constant  OutDataTypeStr=single
  LAS_OverspeedWarningEnableStatus_L : simulink/Logic and Bit Operations/Bitwise Operator  logicop=AND  UseBitMask=on  BitMask=48  BitMaskRealWorld=Stored Integer
  LAS_OverspeedWarningEnableStatus_O : Constant  Value=0  OutDataTypeStr=single
  LAS_OverspeedWarningEnableStatus_S : ArithShift  BitShiftNumber=-4
  LAS_OverspeedWarningEnableStatus_sat : Saturate  UpperLimit=3  LowerLimit=0
  LAS_OverspeedWarningEnableStatus_st : Sum  Inputs=+-
  output1 : Outport
  output2 : Outport  Port=2
  output3 : Outport  Port=3
  output4 : Outport  Port=4
  output5 : Outport  Port=5
  output6 : Outport  Port=6
  output7 : Outport  Port=7
  output8 : Outport  Port=8
  wires:
  LAS_OverspeedWarningEnableStatus/1 -> LAS_OverspeedWarningEnableStatus_sat/1
  LAS_OverspeedWarningEnableStatus_sat/1 -> LAS_OverspeedWarningEnableStatus_st/1
  LAS_OverspeedWarningEnableStatus_O/1 -> LAS_OverspeedWarningEnableStatus_st/2
  LAS_OverspeedWarningEnableStatus_st/1 -> LAS_OverspeedWarningEnableStatus_D/1
  LAS_OverspeedWarningEnableStatus_F/1 -> LAS_OverspeedWarningEnableStatus_D/2
  LAS_OverspeedWarningEnableStatus_D/1 -> LAS_OverspeedWarningEnableStatusRon/1
  LAS_OverspeedWarningEnableStatusRon/1 -> LAS_OverspeedWarningEnableStatus_S/1
  LAS_OverspeedWarningEnableStatus_S/1 -> LAS_OverspeedWarningEnableStatus_1sat/1
  LAS_OverspeedWarningEnableStatus_1sat/1 -> LAS_OverspeedWarningEnableStatus_Convert1/1
  LAS_OverspeedWarningEnableStatus_Convert1/1 -> LAS_OverspeedWarningEnableStatus_L/1
  LAS_OverspeedWarningEnableStatus_L/1 -> LAS_OverspeedWarningEnableStatus_Convert/1
  LAS_OverspeedWarningEnableStatus_Convert/1 -> output4/1
  Constant1/1 -> output1/1
  Constant2/1 -> output2/1
  Constant3/1 -> output3/1
  Constant5/1 -> output5/1
  Constant6/1 -> output6/1
  Constant7/1 -> output7/1
  Constant8/1 -> output8/1

== system VCU_CS75_12_27_test/长安CS75底盘程序，20ms一次/Output/Subsystem/TransmitMessages10/LAS_29D/LAS_OverspeedWarningOffset ==
  LAS_OverspeedWarningOffset : Inport
  Constant{1..5,7..8} (7 alike) : Constant  Value=0  OutDataTypeStr=uint8
  LAS_OverspeedWarningOffsetRon : Rounding  Operator=round
  LAS_OverspeedWarningOffset_1sat : Saturate  UpperLimit=248  LowerLimit=0
  LAS_OverspeedWarningOffset_Convert : DataTypeConversion  OutDataTypeStr=uint8
  LAS_OverspeedWarningOffset_Convert1 : DataTypeConversion  OutDataTypeStr=uint32
  LAS_OverspeedWarningOffset_D : Product  Inputs=*/
  LAS_OverspeedWarningOffset_F : Constant  OutDataTypeStr=single
  LAS_OverspeedWarningOffset_L : simulink/Logic and Bit Operations/Bitwise Operator  logicop=AND  UseBitMask=on  BitMask=248  BitMaskRealWorld=Stored Integer
  LAS_OverspeedWarningOffset_O : Constant  Value=-10  OutDataTypeStr=single
  LAS_OverspeedWarningOffset_S : ArithShift  BitShiftNumber=-3
  LAS_OverspeedWarningOffset_sat : Saturate  UpperLimit=10  LowerLimit=-10
  LAS_OverspeedWarningOffset_st : Sum  Inputs=+-
  output1 : Outport
  output2 : Outport  Port=2
  output3 : Outport  Port=3
  output4 : Outport  Port=4
  output5 : Outport  Port=5
  output6 : Outport  Port=6
  output7 : Outport  Port=7
  output8 : Outport  Port=8
  wires:
  LAS_OverspeedWarningOffset/1 -> LAS_OverspeedWarningOffset_sat/1
  LAS_OverspeedWarningOffset_sat/1 -> LAS_OverspeedWarningOffset_st/1
  LAS_OverspeedWarningOffset_O/1 -> LAS_OverspeedWarningOffset_st/2
  LAS_OverspeedWarningOffset_st/1 -> LAS_OverspeedWarningOffset_D/1
  LAS_OverspeedWarningOffset_F/1 -> LAS_OverspeedWarningOffset_D/2
  LAS_OverspeedWarningOffset_D/1 -> LAS_OverspeedWarningOffsetRon/1
  LAS_OverspeedWarningOffsetRon/1 -> LAS_OverspeedWarningOffset_S/1
  LAS_OverspeedWarningOffset_S/1 -> LAS_OverspeedWarningOffset_1sat/1
  LAS_OverspeedWarningOffset_1sat/1 -> LAS_OverspeedWarningOffset_Convert1/1
  LAS_OverspeedWarningOffset_Convert1/1 -> LAS_OverspeedWarningOffset_L/1
  LAS_OverspeedWarningOffset_L/1 -> LAS_OverspeedWarningOffset_Convert/1
  LAS_OverspeedWarningOffset_Convert/1 -> output6/1
  Constant1/1 -> output1/1
  Constant2/1 -> output2/1
  Constant3/1 -> output3/1
  Constant4/1 -> output4/1
  Constant5/1 -> output5/1
  Constant7/1 -> output7/1
  Constant8/1 -> output8/1

== system VCU_CS75_12_27_test/长安CS75底盘程序，20ms一次/Output/Subsystem/TransmitMessages10/LAS_29D/LAS_RLaneMarkerType ==
  LAS_RLaneMarkerType : Inport
  Constant{1..5,7..8} (7 alike) : Constant  Value=0  OutDataTypeStr=uint8
  LAS_RLaneMarkerTypeRon : Rounding  Operator=round
  LAS_RLaneMarkerType_1sat : Saturate  UpperLimit=7  LowerLimit=0
  LAS_RLaneMarkerType_Convert : DataTypeConversion  OutDataTypeStr=uint8
  LAS_RLaneMarkerType_Convert1 : DataTypeConversion  OutDataTypeStr=uint32
  LAS_RLaneMarkerType_D : Product  Inputs=*/
  LAS_RLaneMarkerType_F : Constant  OutDataTypeStr=single
  LAS_RLaneMarkerType_L : simulink/Logic and Bit Operations/Bitwise Operator  logicop=AND  UseBitMask=on  BitMask=7  BitMaskRealWorld=Stored Integer
  LAS_RLaneMarkerType_O : Constant  Value=0  OutDataTypeStr=single
  LAS_RLaneMarkerType_S : ArithShift
  LAS_RLaneMarkerType_sat : Saturate  UpperLimit=7  LowerLimit=0
  LAS_RLaneMarkerType_st : Sum  Inputs=+-
  output1 : Outport
  output2 : Outport  Port=2
  output3 : Outport  Port=3
  output4 : Outport  Port=4
  output5 : Outport  Port=5
  output6 : Outport  Port=6
  output7 : Outport  Port=7
  output8 : Outport  Port=8
  wires:
  LAS_RLaneMarkerType/1 -> LAS_RLaneMarkerType_sat/1
  LAS_RLaneMarkerType_sat/1 -> LAS_RLaneMarkerType_st/1
  LAS_RLaneMarkerType_O/1 -> LAS_RLaneMarkerType_st/2
  LAS_RLaneMarkerType_st/1 -> LAS_RLaneMarkerType_D/1
  LAS_RLaneMarkerType_F/1 -> LAS_RLaneMarkerType_D/2
  LAS_RLaneMarkerType_D/1 -> LAS_RLaneMarkerTypeRon/1
  LAS_RLaneMarkerTypeRon/1 -> LAS_RLaneMarkerType_S/1
  LAS_RLaneMarkerType_S/1 -> LAS_RLaneMarkerType_1sat/1
  LAS_RLaneMarkerType_1sat/1 -> LAS_RLaneMarkerType_Convert1/1
  LAS_RLaneMarkerType_Convert1/1 -> LAS_RLaneMarkerType_L/1
  LAS_RLaneMarkerType_L/1 -> LAS_RLaneMarkerType_Convert/1
  LAS_RLaneMarkerType_Convert/1 -> output6/1
  Constant1/1 -> output1/1
  Constant2/1 -> output2/1
  Constant3/1 -> output3/1
  Constant4/1 -> output4/1
  Constant5/1 -> output5/1
  Constant7/1 -> output7/1
  Constant8/1 -> output8/1

== system VCU_CS75_12_27_test/长安CS75底盘程序，20ms一次/Output/Subsystem/TransmitMessages10/LAS_29D/LAS_SLASwitchStatus ==
  LAS_SLASwitchStatus : Inport
  Constant{2..8} (7 alike) : Constant  Value=0  OutDataTypeStr=uint8
  LAS_SLASwitchStatusRon : Rounding  Operator=round
  LAS_SLASwitchStatus_1sat : Saturate  UpperLimit=2  LowerLimit=0
  LAS_SLASwitchStatus_Convert : DataTypeConversion  OutDataTypeStr=uint8
  LAS_SLASwitchStatus_Convert1 : DataTypeConversion  OutDataTypeStr=uint32
  LAS_SLASwitchStatus_D : Product  Inputs=*/
  LAS_SLASwitchStatus_F : Constant  OutDataTypeStr=single
  LAS_SLASwitchStatus_L : simulink/Logic and Bit Operations/Bitwise Operator  logicop=AND  UseBitMask=on  BitMask=2  BitMaskRealWorld=Stored Integer
  LAS_SLASwitchStatus_O : Constant  Value=0  OutDataTypeStr=single
  LAS_SLASwitchStatus_S : ArithShift  BitShiftNumber=-1
  LAS_SLASwitchStatus_sat : Saturate  UpperLimit=1  LowerLimit=0
  LAS_SLASwitchStatus_st : Sum  Inputs=+-
  output1 : Outport
  output2 : Outport  Port=2
  output3 : Outport  Port=3
  output4 : Outport  Port=4
  output5 : Outport  Port=5
  output6 : Outport  Port=6
  output7 : Outport  Port=7
  output8 : Outport  Port=8
  wires:
  LAS_SLASwitchStatus/1 -> LAS_SLASwitchStatus_sat/1
  LAS_SLASwitchStatus_sat/1 -> LAS_SLASwitchStatus_st/1
  LAS_SLASwitchStatus_O/1 -> LAS_SLASwitchStatus_st/2
  LAS_SLASwitchStatus_st/1 -> LAS_SLASwitchStatus_D/1
  LAS_SLASwitchStatus_F/1 -> LAS_SLASwitchStatus_D/2
  LAS_SLASwitchStatus_D/1 -> LAS_SLASwitchStatusRon/1
  LAS_SLASwitchStatusRon/1 -> LAS_SLASwitchStatus_S/1
  LAS_SLASwitchStatus_S/1 -> LAS_SLASwitchStatus_1sat/1
  LAS_SLASwitchStatus_1sat/1 -> LAS_SLASwitchStatus_Convert1/1
  LAS_SLASwitchStatus_Convert1/1 -> LAS_SLASwitchStatus_L/1
  LAS_SLASwitchStatus_L/1 -> LAS_SLASwitchStatus_Convert/1
  LAS_SLASwitchStatus_Convert/1 -> output1/1
  Constant2/1 -> output2/1
  Constant3/1 -> output3/1
  Constant4/1 -> output4/1
  Constant5/1 -> output5/1
  Constant6/1 -> output6/1
  Constant7/1 -> output7/1
  Constant8/1 -> output8/1
